simulink subsystem "MyPieroAjusteRuedas"  (R2022b)
settings: Solver=VariableStepAuto  StartTime=0.0  StopTime=10.0  RelTol=1e-3
settings Model: Creator=Usuario  LastModifiedBy=Usuario

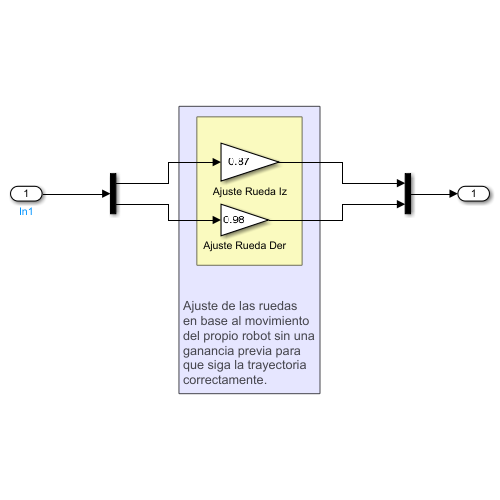
[thumbnail: Simulink's stored preview of the top-level diagram]
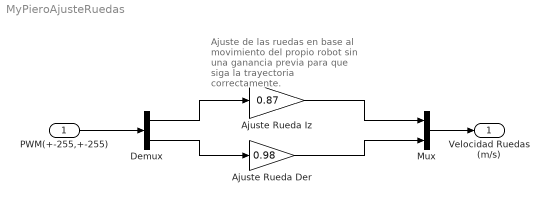
== system MyPieroAjusteRuedas ==
  note: Ajuste de las ruedas
      | en base al movimiento
      | del propio robot sin una
      | ganancia previa para
      | que siga la trayectoria
      | correctamente.
  PWM(+-255,+-255) : Inport
  Ajuste Rueda Der : Gain  Gain=0.98
  Ajuste Rueda Iz : Gain  Gain=0.87
  Demux : Demux  Outputs=2
  Mux : Mux  Inputs=2
  Velocidad Ruedas (m/s) : Outport
  wires:
  PWM(+-255,+-255)/1 -> Demux/1
  Demux/2 -> Ajuste Rueda Der/1
  Demux/1 -> Ajuste Rueda Iz/1
  Ajuste Rueda Iz/1 -> Mux/1
  Ajuste Rueda Der/1 -> Mux/2
  Mux/1 -> Velocidad Ruedas (m/s)/1
